simulink model "ripHardware"  (R2024a)
settings: Solver=FixedStepAuto  StartTime=0.0  StopTime=30  FixedStep=0.01  RelTol=1e-3
undefined symbols (not defined in the file or in its folder): daq
libraries: daqlib x1, simulink_extras x1, fuzblock x1
settings Model: Creator=Ali_Omran  LastModifiedBy=Ali_Omran

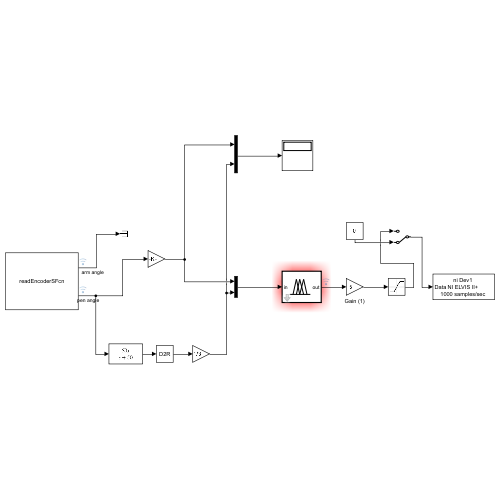
[thumbnail: Simulink's stored preview of the top-level diagram]
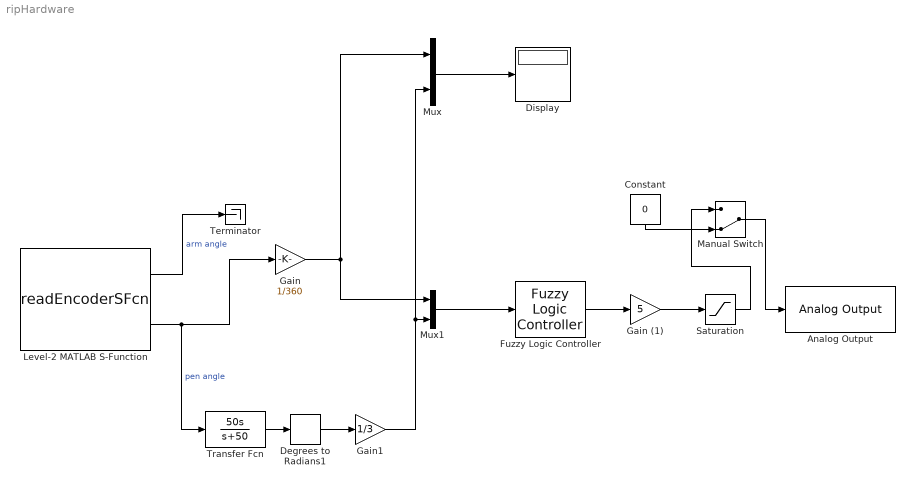
== system ripHardware ==
  Analog Output : daqlib/Analog Output  DeviceMenu=(none)  Device=ni Dev1 (NI ELVIS II+)  ObjConstructor=daq.createSession('ni')  NChannelsSelected=1  Channels=1$ao0$$Dev1$1$2$N/A$#0$ao1$$Dev1$1$2$N/A$#  NPorts=1 for all channels  SampleRate=1000  ActualRate=1000
  Constant : Constant  Value=0
  Degrees to Radians1 : simulink_extras/Transformations/Degrees to Radians
  Display : Display
  Fuzzy Logic Controller : fuzblock/Fuzzy Logic  Controller  FIS=mamT1_RIP_Stabilize2  OutputSampleNumber=101  DataType=double  FuzzifiedInputs=off  RuleFiringStrengths=off  RuleOutputs=off  AggregatedOutputs=off  SimulateUsing=Interpreted execution  OutOfRangeInputValueMessage=warning  NoRuleFiredMessage=warning  EmptyOutputFuzzySetMessage=warning
  Gain : Gain  Gain=1/360
  Gain (1) : Gain  Gain=5
  Gain1 : Gain  Gain=1/3
  Level-2 MATLAB S-Function : M-S-Function  FunctionName=readEncoderSFcn
  Manual Switch : ManualSwitch  CurrentSetting=0
  Mux : Mux  Inputs=2
  Mux1 : Mux  Inputs=2
  Saturation : Saturate  UpperLimit=5  LowerLimit=-5
  Terminator : Terminator
  Transfer Fcn : TransferFcn  Numerator=[50 0]  Denominator=[1 50]
  wires:
  Level-2 MATLAB S-Function/2 -> Gain/1, Transfer Fcn/1  "pen angle"
  Mux/1 -> Display/1
  Level-2 MATLAB S-Function/1 -> Terminator/1  "arm angle"
  Degrees to Radians1/1 -> Gain1/1
  Gain (1)/1 -> Saturation/1
  Fuzzy Logic Controller/1 -> Gain (1)/1
  Gain1/1 -> Mux/2, Mux1/2
  Gain/1 -> Mux1/1, Mux/1
  Mux1/1 -> Fuzzy Logic Controller/1
  Manual Switch/1 -> Analog Output/1
  Saturation/1 -> Manual Switch/1
  Constant/1 -> Manual Switch/2
  Transfer Fcn/1 -> Degrees to Radians1/1
